simulink model "matlab_combined_demo_model"  (R2022b)
settings: Solver=ode4  StartTime=0.0  StopTime=inf  FixedStep=0.003  RelTol=1e-3
values from neighbouring files (symbols this model uses):
  A1 = 0    [load_quadrotor_simulink_combined_model.m]    (also in load_quadrotor_simulink_physics_model.m; load_quadtiltrotor_simulink_physics_model.m = 0.007)
  Apolar = 0    [load_quadrotor_simulink_combined_model.m]    (also in load_quadrotor_simulink_physics_model.m; load_quadtiltrotor_simulink_physics_model.m = 0.057)
  CD0 = 0    [load_quadrotor_simulink_combined_model.m]    (also in load_quadrotor_simulink_physics_model.m; load_quadtiltrotor_simulink_physics_model.m = 0.022)
  chord = 1    [load_quadrotor_simulink_combined_model.m]    (also in load_quadrotor_simulink_physics_model.m; load_quadtiltrotor_simulink_physics_model.m = 0.351342)
  CL0 = 0    [load_quadrotor_simulink_combined_model.m]    (also in load_quadrotor_simulink_physics_model.m; load_quadtiltrotor_simulink_physics_model.m = 0.38)
  CLa = 0    [load_quadrotor_simulink_combined_model.m]    (also in load_quadrotor_simulink_physics_model.m; load_quadtiltrotor_simulink_physics_model.m = 18.5)
  CLa_dot = 0    [load_quadrotor_simulink_combined_model.m]    (also in load_quadrotor_simulink_physics_model.m; load_quadtiltrotor_simulink_physics_model.m = 2.64)
  Clb = 0    [load_quadrotor_simulink_combined_model.m]    (also in load_quadrotor_simulink_physics_model.m; load_quadtiltrotor_simulink_physics_model.m)
  ClDa = 0    [load_quadrotor_simulink_combined_model.m]    (also in load_quadrotor_simulink_physics_model.m; load_quadtiltrotor_simulink_physics_model.m = 0.1695)
  CLDe = 0    [load_quadrotor_simulink_combined_model.m]    (also in load_quadrotor_simulink_physics_model.m; load_quadtiltrotor_simulink_physics_model.m)
  CLDf = 0    [load_quadrotor_simulink_combined_model.m]    (also in load_quadrotor_simulink_physics_model.m; load_quadtiltrotor_simulink_physics_model.m = 0.4)
  ClDr = 0    [load_quadrotor_simulink_combined_model.m]    (also in load_quadrotor_simulink_physics_model.m; load_quadtiltrotor_simulink_physics_model.m)
  Clp = 0    [load_quadrotor_simulink_combined_model.m]    (also in load_quadrotor_simulink_physics_model.m; load_quadtiltrotor_simulink_physics_model.m)
  CLq = 0    [load_quadrotor_simulink_combined_model.m]    (also in load_quadrotor_simulink_physics_model.m; load_quadtiltrotor_simulink_physics_model.m = 7.4)
  Clr = 0    [load_quadrotor_simulink_combined_model.m]    (also in load_quadrotor_simulink_physics_model.m; load_quadtiltrotor_simulink_physics_model.m)
  Cm0 = 0    [load_quadrotor_simulink_combined_model.m]    (also in load_quadrotor_simulink_physics_model.m; load_quadtiltrotor_simulink_physics_model.m)
  Cma = 0    [load_quadrotor_simulink_combined_model.m]    (also in load_quadrotor_simulink_physics_model.m; load_quadtiltrotor_simulink_physics_model.m)
  CmDe = 0    [load_quadrotor_simulink_combined_model.m]    (also in load_quadrotor_simulink_physics_model.m; load_quadtiltrotor_simulink_physics_model.m = -3.2)
  CmDf = 0    [load_quadrotor_simulink_combined_model.m]    (also in load_quadrotor_simulink_physics_model.m; load_quadtiltrotor_simulink_physics_model.m)
  Cmq = 0    [load_quadrotor_simulink_combined_model.m]    (also in load_quadrotor_simulink_physics_model.m; load_quadtiltrotor_simulink_physics_model.m)
  Cnb = 0    [load_quadrotor_simulink_combined_model.m]    (also in load_quadrotor_simulink_physics_model.m; load_quadtiltrotor_simulink_physics_model.m)
  CnDa = 0    [load_quadrotor_simulink_combined_model.m]    (also in load_quadrotor_simulink_physics_model.m; load_quadtiltrotor_simulink_physics_model.m = -0.023)
  CnDr = 0    [load_quadrotor_simulink_combined_model.m]    (also in load_quadrotor_simulink_physics_model.m; load_quadtiltrotor_simulink_physics_model.m)
  Cnp = 0    [load_quadrotor_simulink_combined_model.m]    (also in load_quadrotor_simulink_physics_model.m; load_quadtiltrotor_simulink_physics_model.m = -0.0889)
  Cnr = 0    [load_quadrotor_simulink_combined_model.m]    (also in load_quadrotor_simulink_physics_model.m; load_quadtiltrotor_simulink_physics_model.m = -0.19997)
  cross_section_area = 1    [load_quadrotor_simulink_combined_model.m]    (also in load_quadrotor_simulink_physics_model.m; load_quadtiltrotor_simulink_physics_model.m = 9.5)
  CYb = 0    [load_quadrotor_simulink_combined_model.m]    (also in load_quadrotor_simulink_physics_model.m; load_quadtiltrotor_simulink_physics_model.m = -1.098)
  CYDr = 0    [load_quadrotor_simulink_combined_model.m]    (also in load_quadrotor_simulink_physics_model.m; load_quadtiltrotor_simulink_physics_model.m = 0.143)
  drag_coeff_angular = -0.5    [load_quadrotor_simulink_combined_model.m]    (also in load_quadrotor_simulink_physics_model.m; load_quadtiltrotor_simulink_physics_model.m = 0.2)
  drag_coeff_linear = -0.5    [load_quadrotor_simulink_combined_model.m]    (also in load_quadrotor_simulink_physics_model.m; load_quadtiltrotor_simulink_physics_model.m = 0.2)
  elarm = 0    [load_quadrotor_simulink_combined_model.m]    (also in load_quadrotor_simulink_physics_model.m; load_quadtiltrotor_simulink_physics_model.m = 0.121)
  enable_FW_forces = 0    [load_quadrotor_simulink_combined_model.m]    (also in load_quadrotor_simulink_physics_model.m; load_quadtiltrotor_simulink_physics_model.m = 1)
  initial_rpy = [0, 0, 0]    [load_quadrotor_simulink_combined_model.m]    (also in load_quadrotor_simulink_physics_model.m; load_quadtiltrotor_simulink_physics_model.m)
  initial_xyz = [0, 0, -4]    [load_quadrotor_simulink_combined_model.m]    (also in load_quadrotor_simulink_physics_model.m; load_quadtiltrotor_simulink_physics_model.m = [2, 3, -4])
  mass = 1    [load_quadrotor_simulink_combined_model.m]    (also in load_quadrotor_simulink_physics_model.m; load_quadtiltrotor_simulink_physics_model.m = 10)
  span = 0    [load_quadrotor_simulink_combined_model.m]    (also in load_quadrotor_simulink_physics_model.m; load_quadtiltrotor_simulink_physics_model.m = 2.795)
libraries: aerolibutil x6, simulink x4, vrlib x4, sharedtransform x2, aerolibasang x2, shared6dof x1, matrix_library x1
(part 1 of 2)
settings Model: Creator=edufford  LastModifiedBy=edufford
settings DebuggingCC: UnconnectedInputMsg=warning  UnconnectedOutputMsg=warning  UnconnectedLineMsg=warning
settings ModelReferenceCC: EnableRefExpFcnMdlSchedulingChecks=on
settings RTWCC: DLArmComputeVersion=19.05

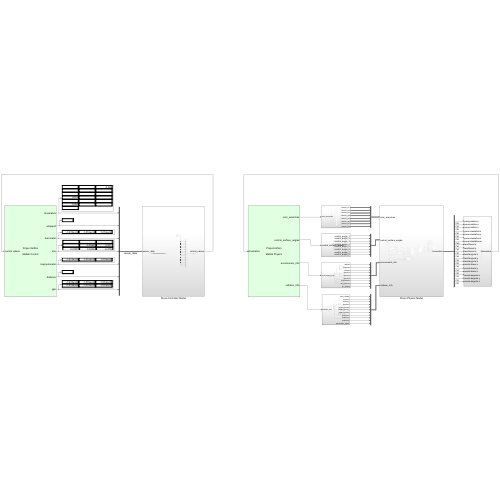
[thumbnail: Simulink's stored preview of the top-level diagram]
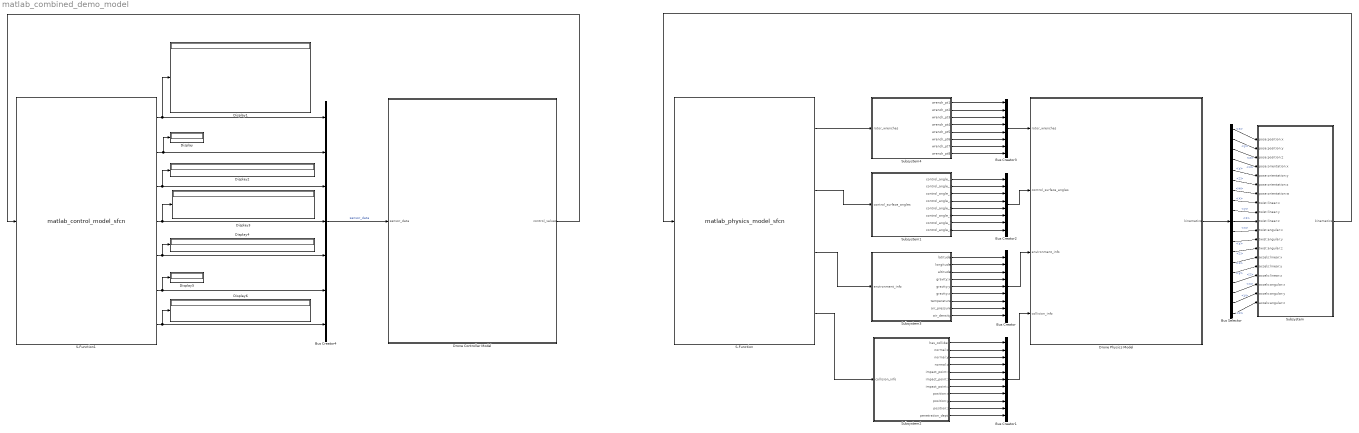
== system matlab_combined_demo_model ==
  Bus Creator : BusCreator  Inputs=9
  Bus Creator1 : BusCreator  Inputs=11
  Bus Creator2 : BusCreator  Inputs=8
  Bus Creator3 : BusCreator  Inputs=8
  Bus Creator4 : BusCreator  Inputs=7
  Bus Selector : BusSelector  OutputSignals=pose.position.x,pose.position.y,pose.position.z,pose.orientation.x,pose.orientation.y,pose.orientation.z,pose.orientation.w,twist.linear.x,twist.linear.y,twist.linear.z,twist.angular.x,twist.angular.y,twist.angular.z,accels.linear.x,accels.linear.y,accels.linear.z,accels.angular.x,accels.angular.y,accels.angular.z
  Display{,1..6} (7 alike) : Display
  Drone Controller Model : Subsystem
  Drone Physics Model : Subsystem
  S-Function : S-Function  Priority=10  FunctionName=matlab_physics_model_sfcn  Parameters=hostname,portnumber,timestep  SFunctionDeploymentMode=off  EnableBusSupport=off  mask{hostname=*, portnumber=8999, timestep=0.003}
      mask prompts: hostname "Host name:"; portnumber "Port number:"; timestep "AirSim time step:"
      mask Display:
      | disp("Project AirSim\n\n")
      | disp("\n\nMatlab Physics")
      | port_label('input',1,'kinematics')
      | port_label('output',1,'rotor_wrenches')
      | port_label('output',2,'control_surface_angles')
      | port_label('output',3,'environment_info')
      | port_label('output',4,'collision_info')
  S-Function1 : S-Function  Priority=20  FunctionName=matlab_control_model_sfcn  Parameters=hostname,portnumber,timestep  SFunctionDeploymentMode=off  EnableBusSupport=off  mask{hostname=*, portnumber=8998, timestep=0.003}
      mask prompts: hostname "Host name:"; portnumber "Port number:"; timestep "AirSim time step:"
      mask Display:
      | disp("Project AirSim\n\n")
      | disp("\n\nMatlab Control")
      | port_label('input',1,'control values')
      | port_label('output',1,'kinematics')
      | port_label('output',2,'airspeed')
      | port_label('output',3,'barometer')
      | port_label('output',4,'imu')
      | port_label('output',5,'magnetometer')
      | port_label('output',6,'distance')
      | port_label('output',7,'gps')
  Subsystem : Subsystem
  Subsystem1 : Subsystem
  Subsystem2 : Subsystem
  Subsystem3 : Subsystem
  Subsystem4 : Subsystem
  wires:
  Subsystem/1(kinematics) -> S-Function/1
  S-Function/4 -> Subsystem2/1(collision_info)
  Subsystem2/2(normal:x) -> Bus Creator1/2
  Subsystem2/5(impact_point:x) -> Bus Creator1/5
  Subsystem2/3(normal:y) -> Bus Creator1/3
  Subsystem2/4(normal:z) -> Bus Creator1/4
  Subsystem2/6(impact_point:y) -> Bus Creator1/6
  Subsystem2/7(impact_point:z) -> Bus Creator1/7
  Subsystem2/8(position:x) -> Bus Creator1/8
  Subsystem2/9(position:y) -> Bus Creator1/9
  Subsystem2/10(position:z) -> Bus Creator1/10
  Subsystem2/11(penetration_depth) -> Bus Creator1/11
  S-Function/3 -> Subsystem3/1(environment_info)
  Subsystem3/2(longitude) -> Bus Creator/2
  Subsystem3/3(altitude) -> Bus Creator/3
  Subsystem3/4(gravity:x) -> Bus Creator/4
  Subsystem3/5(gravity:y) -> Bus Creator/5
  Subsystem3/6(gravity:z) -> Bus Creator/6
  Subsystem3/7(temperature) -> Bus Creator/7
  Subsystem3/8(air_pressure) -> Bus Creator/8
  Subsystem3/9(air_density) -> Bus Creator/9
  Subsystem3/1(latitude) -> Bus Creator/1
  Bus Creator/1 -> Drone Physics Model/3(environment_info)
  Subsystem2/1(has_collided) -> Bus Creator1/1
  Bus Creator1/1 -> Drone Physics Model/4(collision_info)
  S-Function/1 -> Subsystem4/1(rotor_wrenches)
  Subsystem4/1(wrench_pt1) -> Bus Creator3/1
  Subsystem4/2(wrench_pt2) -> Bus Creator3/2
  Subsystem4/3(wrench_pt3) -> Bus Creator3/3
  Subsystem4/4(wrench_pt4) -> Bus Creator3/4
  Bus Creator3/1 -> Drone Physics Model/1(rotor_wrenches)
  Drone Physics Model/1(kinematics) -> Bus Selector/1
  Bus Selector/1 -> Subsystem/1(pose:position:x)  "<x>"
  Bus Selector/2 -> Subsystem/2(pose:position:y)  "<y>"
  Bus Selector/3 -> Subsystem/3(pose:position:z)  "<z>"
  Bus Selector/4 -> Subsystem/4(pose:orientation:x)  "<x>"
  Bus Selector/5 -> Subsystem/5(pose:orientation:y)  "<y>"
  Bus Selector/6 -> Subsystem/6(pose:orientation:z)  "<z>"
  Bus Selector/7 -> Subsystem/7(pose:orientation:w)  "<w>"
  Bus Selector/8 -> Subsystem/8(twist:linear:x)  "<x>"
  Bus Selector/9 -> Subsystem/9(twist:linear:y)  "<y>"
  Bus Selector/10 -> Subsystem/10(twist:linear:z)  "<z>"
  Bus Selector/11 -> Subsystem/11(twist:angular:x)  "<x>"
  Bus Selector/12 -> Subsystem/12(twist:angular:y)  "<y>"
  Bus Selector/13 -> Subsystem/13(twist:angular:z)  "<z>"
  Bus Selector/14 -> Subsystem/14(accels:linear:x)  "<x>"
  Bus Selector/15 -> Subsystem/15(accels:linear:y)  "<y>"
  Bus Selector/16 -> Subsystem/16(accels:linear:z)  "<z>"
  Bus Selector/17 -> Subsystem/17(accels:angular:x)  "<x>"
  Bus Selector/18 -> Subsystem/18(accels:angular:y)  "<y>"
  Bus Selector/19 -> Subsystem/19(accels:angular:z)  "<z>"
  Bus Creator2/1 -> Drone Physics Model/2(control_surface_angles)
  Subsystem1/1(control_angle_1) -> Bus Creator2/1
  Subsystem1/2(control_angle_2) -> Bus Creator2/2
  Subsystem1/3(control_angle_3) -> Bus Creator2/3
  S-Function/2 -> Subsystem1/1(control_surface_angles)
  Subsystem4/5(wrench_pt5) -> Bus Creator3/5
  Subsystem4/6(wrench_pt6) -> Bus Creator3/6
  Subsystem4/7(wrench_pt7) -> Bus Creator3/7
  Subsystem4/8(wrench_pt8) -> Bus Creator3/8
  Subsystem1/4(control_angle_4) -> Bus Creator2/4
  Subsystem1/5(control_angle_5) -> Bus Creator2/5
  Subsystem1/6(control_angle_6) -> Bus Creator2/6
  Subsystem1/7(control_angle_7) -> Bus Creator2/7
  Subsystem1/8(control_angle_8) -> Bus Creator2/8
  Drone Controller Model/1(control_values) -> S-Function1/1
  S-Function1/1 -> Display1/1, Bus Creator4/1
  S-Function1/2 -> Bus Creator4/2, Display/1
  S-Function1/3 -> Display2/1, Bus Creator4/3
  S-Function1/4 -> Display3/1, Bus Creator4/4
  S-Function1/5 -> Display4/1, Bus Creator4/5
  S-Function1/6 -> Display5/1, Bus Creator4/6
  S-Function1/7 -> Display6/1, Bus Creator4/7
  Bus Creator4/1 -> Drone Controller Model/1(sensor_data)  "sensor_data"

== system matlab_combined_demo_model/Drone Controller Model ==
  sensor_data : Inport
  Mux : Mux  Inputs=16
  Repeating Sequence : simulink/Sources/Repeating Sequence  rep_seq_t=[0 5 10]  rep_seq_y=[0 1 0]
  Terminator : Terminator
  control_values : Outport
  wires:
  Repeating Sequence/1 -> Mux/1, Mux/2, Mux/3, Mux/7, Mux/8, Mux/9, Mux/10, Mux/11, Mux/14, Mux/15, Mux/16, Mux/13, Mux/12, Mux/6, Mux/5, Mux/4
  Mux/1 -> control_values/1
  sensor_data/1 -> Terminator/1

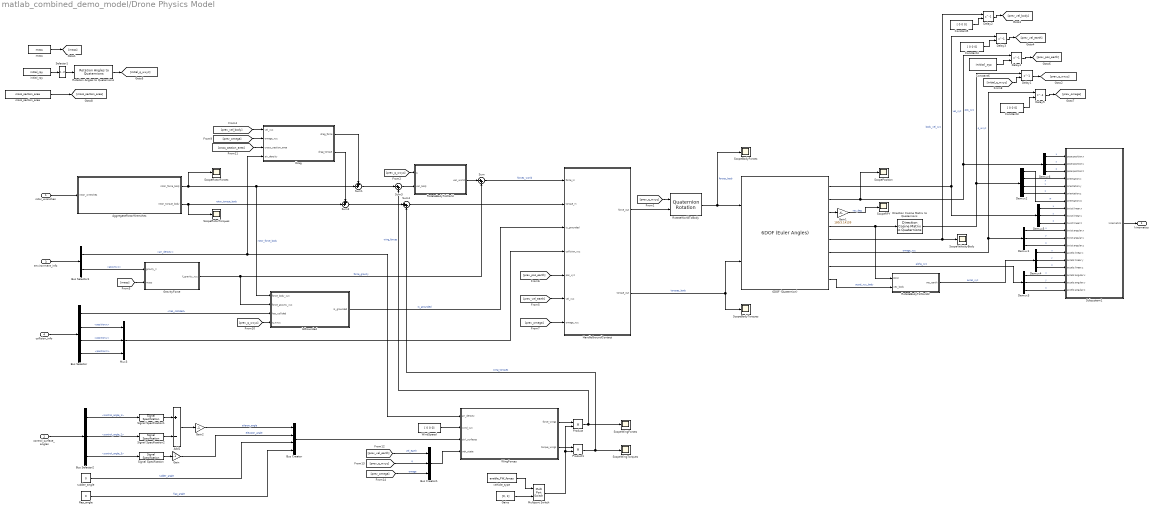
== system matlab_combined_demo_model/Drone Physics Model ==
  rotor_wrenches : Inport
  control_surface_angles : Inport  Port=2
  environment_info : Inport  Port=3
  collision_info : Inport  Port=4
  6DOF (Quaternion) : shared6dof/6DOF (Euler Angles)  units=Metric (MKS)  mtype=Fixed  rep=Quaternion  xme_0=initial_xyz  Vm_0=initial_vel_xyz  eul_0=initial_rpy  pm_0=initial_ang_rot_xyz  mass_0=mass  mass_e=0.5  mass_f=2.0  inertia=inertia  inertia_e=eye(3)  inertia_f=2*eye(3)  k_quat=1.0  vre_flag=on  abi_flag=off  aMode=0  xme_statename=''  Vm_statename=''  eul_statename=''  quat_statename=''  pm_statename=''  mass_statename=''
  Add1 : Sum  Inputs=+-
  AggregateRotorWrenches : Subsystem
  Bus Creator : BusCreator  Inputs=4
  Bus Creator1 : BusCreator  Inputs=3
  Bus Selector : BusSelector  OutputSignals=has_collided,position:x,position:y,position:z
  Bus Selector1 : BusSelector  OutputSignals=air_density,gravity:z
  Bus Selector2 : BusSelector  OutputSignals=control_angle_1,control_angle_2,control_angle_3
  Constant3 : Constant  Value=[ 0 0 0]
      settings: AttributesFormatString=%<Value>
  Constant4 : Constant  Value=[ 0 0 0]
      settings: AttributesFormatString=%<Value>
  Constant5 : Constant  Value=[ 0 0 0]
      settings: AttributesFormatString=%<Value>
  Constant6 : Constant  Value=initial_xyz
      settings: AttributesFormatString=%<Value>
  Delay{1..5} (5 alike) : Delay  DelayLength=1  InitialConditionSource=Input port  InitialCondition=0
      settings: InputPortMap=u0,p4
  Demux{1,3..6} (5 alike) : Demux  Outputs=3
  Demux2 : Demux
  Direction Cosine Matrix to Quaternions : sharedtransform/Direction Cosine Matrix  to Quaternions  aMode=0  action=None  tolerance=eps(2)
  Drag : Subsystem
  Gain : Gain  Gain=-1
  Gain1 : Gain  Gain=180/3.14159
  Gain2 : Gain  Gain=-1
  Gains : Constant  Value=[0, 1]
  GravityForce : Subsystem
  HandleGroundContact : Subsystem
  IsGrounded : Subsystem
  Multiport Switch : MultiPortSwitch  DataPortOrder=Zero-based contiguous  Inputs=1  zeroidx=on  SaturateOnIntegerOverflow=off  InputSameDT=off
  Mux3 : Mux  Inputs=3
  Product : Product
  Product1 : Product
  RotateBodyToWorld : Subsystem
  RotateBodyToWorld2 : Subsystem
  RotateWorldToBody : aerolibutil/Quaternion Rotation
  Rotation Angles to Quaternions : sharedtransform/Rotation Angles to Quaternions  rotationOrder=ZYX  aMode=aMode
  ScopeBodyForces : Scope
  ScopeBodyTorques : Scope
  ScopePosition : Scope
  ScopeRPY : Scope
  ScopeRotorForces : Scope
  ScopeRotorTorques : Scope
  ScopeVelocityBody : Scope
  ScopeWingForces : Scope
  ScopeWingTorques : Scope
  Selector1 : Selector  InputPortWidth=3  IndexOptions=Index vector (dialog)  Indices=[3 2 1]  OutputSizes=1
  Signal Specification : SignalSpecification  Unit=rad
  Signal Specification1 : SignalSpecification  Unit=rad
  Signal Specification2 : SignalSpecification  Unit=rad
  Subsystem1 : Subsystem
  Sum : Sum  Inputs=|++
  Sum1 : Sum  Inputs=++|
  Sum2 : Sum  Inputs=++|
  Sum3 : Sum  Inputs=|++
  Sum4 : Sum  Inputs=|++
  WindSpeed : Constant  Value=[ 0 0 0]
      settings: AttributesFormatString=%<Value>
  WingForces : Subsystem
  cross_section_area : Constant  Value=cross_section_area
  flap_angle : Constant  Value=0
  initial_rpy : Constant  Value=initial_rpy
  mass : Constant  Value=mass
  rudder_angle : Constant  Value=0
  vehicle_type : Constant  Value=enable_FW_forces
  kinematics : Outport
  wires:
  collision_info/1 -> Bus Selector/1
  environment_info/1 -> Bus Selector1/1
  rotor_wrenches/1 -> AggregateRotorWrenches/1(rotor_wrenches)
  Subsystem1/1(kinematics) -> kinematics/1
  Demux2/2 -> Subsystem1/4(orientation:x)  "x"
  Demux2/3 -> Subsystem1/5(orientation:y)  "y"
  Demux2/4 -> Subsystem1/6(orientation:z)  "z"
  Bus Selector/1 -> IsGrounded/3(has_collided)  "<has_collided>"
  Demux2/1 -> Subsystem1/7(orientation:w)  "w"
  Demux1/1 -> Subsystem1/11(twist:angular:x)  "x"
  Demux1/2 -> Subsystem1/12(twist:angular:y)  "y"
  Demux1/3 -> Subsystem1/13(twist:angular:z)  "z"
  Demux3/1 -> Subsystem1/17(accels:angular:x)  "x"
  Demux3/2 -> Subsystem1/18(accels:angular:y)  "y"
  Demux3/3 -> Subsystem1/19(accels:angular:z)  "z"
  initial_rpy/1 -> Selector1/1
  IsGrounded/1(is_grounded) -> HandleGroundContact/3(is_grounded)  "is_grounded"
  Bus Selector/4 -> Mux3/3  "<position:z>"
  [initial_q_wxyz] -> Delay1/2
  Demux4/1 -> Subsystem1/14(accels:linear:x)  "x"
  Demux4/2 -> Subsystem1/15(accels:linear:y)  "y"
  Demux4/3 -> Subsystem1/16(accels:linear:z)  "z"
  Demux5/1 -> Subsystem1/8(twist:linear:x)  "x"
  Demux5/2 -> Subsystem1/9(twist:linear:y)  "y"
  Demux5/3 -> Subsystem1/10(twist:linear:z)  "z"
  Demux6/1 -> Subsystem1/1(pose:position:x)  "x"
  Demux6/2 -> Subsystem1/2(pose:position:y)  "y"
  Demux6/3 -> Subsystem1/3(pose:position:z)  "z"
  6DOF (Quaternion)/1 -> Demux5/1, Delay3/1  "vel_xyz"
  6DOF (Quaternion)/3 -> Gain1/1
  6DOF (Quaternion)/4 -> RotateBodyToWorld2/1(DCM), Direction Cosine Matrix to Quaternions/1
  6DOF (Quaternion)/7 -> Demux3/1  "alpha_xyz"
  mass/1 -> [mass]
  6DOF (Quaternion)/2 -> Demux6/1, Delay4/1, ScopePosition/1  "pos_xyz"
  Direction Cosine Matrix to Quaternions/1 -> Demux2/1, Delay1/1  "q_wxyz"
  6DOF (Quaternion)/8 -> RotateBodyToWorld2/2(vec_body)  "accel_xyz_body"
  RotateBodyToWorld2/1(vec_earth) -> Demux4/1  "accel_xyz"
  Rotation Angles to Quaternions/1 -> [initial_q_wxyz]
  Selector1/1 -> Rotation Angles to Quaternions/1
  Delay1/1 -> [prev_q_wxyz]
  [prev_q_wxyz] -> RotateWorldToBody/1
  Delay2/1 -> [prev_vel_body]
  [prev_vel_body] -> Drag/1(vel_xyz)
  Delay3/1 -> [prev_vel_earth]
  [prev_vel_earth] -> HandleGroundContact/6(vel_xyz)
  Delay4/1 -> [prev_pos_earth]
  [prev_pos_earth] -> HandleGroundContact/5(pos_xyz)
  Delay5/1 -> [prev_omega]
  [prev_omega] -> HandleGroundContact/7(omega_xyz)
  Bus Selector/3 -> Mux3/2  "<position:y>"
  Bus Selector/2 -> Mux3/1  "<position:x>"
  Mux3/1 -> HandleGroundContact/4(collision_xyz)
  GravityForce/1(f_gravity_xyz) -> IsGrounded/2(force_gravity_xyz), Sum/2  "force_gravity"
  Bus Selector1/2 -> GravityForce/1(gravity_z)  "<gravity:z>"
  [mass] -> GravityForce/2(mass)
  [prev_q_wxyz] -> RotateBodyToWorld/1(q)
  RotateBodyToWorld/1(vec_world) -> Sum/1
  [prev_omega] -> Drag/2(omega_xyz)
  HandleGroundContact/2(torque_out) -> 6DOF (Quaternion)/2, ScopeBodyTorques/1  "torques_body"
  RotateWorldToBody/1 -> 6DOF (Quaternion)/1, ScopeBodyForces/1  "forces_body"
  HandleGroundContact/1(force_out) -> RotateWorldToBody/2
  Sum/1 -> HandleGroundContact/1(force_in)  "forces_world"
  Drag/2(drag_torque) -> Sum2/1
  Drag/1(drag_force) -> Sum1/1
  Sum1/1 -> Sum3/1
  [prev_q_wxyz] -> IsGrounded/4(q_wxyz)
  Sum4/1 -> HandleGroundContact/2(torque_in)
  Gain1/1 -> ScopeRPY/1  "rpy_deg"
  Bus Selector1/1 -> Drag/4(air_density), WingForces/1(air_density)  "<air_density>"
  [cross_section_area] -> Drag/3(cross_section_area)
  control_surface_angles/1 -> Bus Selector2/1
  Bus Selector2/1 -> Signal Specification1/1  "<control_angle_1>"
  Bus Selector2/2 -> Signal Specification2/1  "<control_angle_2>"
  Bus Selector2/3 -> Signal Specification/1  "<control_angle_3>"
  Signal Specification1/1 -> Add1/1
  Signal Specification2/1 -> Add1/2
  flap_angle/1 -> Bus Creator/4  "flap_angle"
  Sum3/1 -> RotateBodyToWorld/2(vec_body)
  Sum2/1 -> Sum4/1
  Constant3/1 -> Delay5/2
  Constant4/1 -> Delay3/2
  Constant5/1 -> Delay2/2
  Constant6/1 -> Delay4/2
  Bus Creator/1 -> WingForces/3(ctrl_surfaces)
  [prev_vel_earth] -> Bus Creator1/1  "vel_earth"
  [prev_q_wxyz] -> Bus Creator1/2  "q"
  [prev_omega] -> Bus Creator1/3  "omega"
  Bus Creator1/1 -> WingForces/4(veh_state)
  WindSpeed/1 -> WingForces/2(wind_xyz)
  Signal Specification/1 -> Gain/1
  Add1/1 -> Gain2/1
  6DOF (Quaternion)/6 -> Demux1/1, Delay5/1  "omega_xyz"
  6DOF (Quaternion)/5 -> ScopeVelocityBody/1, Delay2/1  "body_vel_xyz"
  rudder_angle/1 -> Bus Creator/3  "rudder_angle"
  Gain/1 -> Bus Creator/2  "elevator_angle"
  Gain2/1 -> Bus Creator/1  "aileron_angle"
  cross_section_area/1 -> [cross_section_area]
  vehicle_type/1 -> Multiport Switch/1
  Gains/1 -> Multiport Switch/2
  AggregateRotorWrenches/2(rotor_torque_body) -> Sum2/2, ScopeRotorTorques/1  "rotor_torque_body"
  AggregateRotorWrenches/1(rotor_force_body) -> Sum1/2, IsGrounded/1(force_body_xyz), ScopeRotorForces/1  "rotor_force_body"
  WingForces/1(force_wings) -> Product/1
  Product/1 -> Sum3/2, ScopeWingForces/1  "wing_forces"
  WingForces/2(torque_wings) -> Product1/1
  Product1/1 -> ScopeWingTorques/1, Sum4/2  "wing_torques"
  Multiport Switch/1 -> Product1/2, Product/2

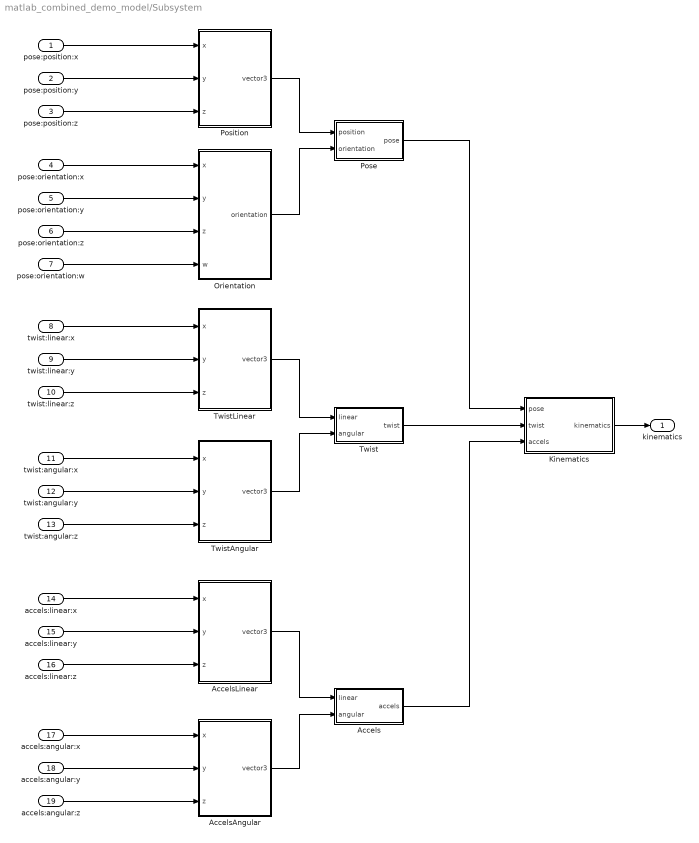
== system matlab_combined_demo_model/Subsystem ==
  pose:position:x : Inport
  pose:position:y : Inport  Port=2
  pose:position:z : Inport  Port=3
  pose:orientation:x : Inport  Port=4
  pose:orientation:y : Inport  Port=5
  pose:orientation:z : Inport  Port=6
  pose:orientation:w : Inport  Port=7
  twist:linear:x : Inport  Port=8
  twist:linear:y : Inport  Port=9
  twist:linear:z : Inport  Port=10
  twist:angular:x : Inport  Port=11
  twist:angular:y : Inport  Port=12
  twist:angular:z : Inport  Port=13
  accels:linear:x : Inport  Port=14
  accels:linear:y : Inport  Port=15
  accels:linear:z : Inport  Port=16
  accels:angular:x : Inport  Port=17
  accels:angular:y : Inport  Port=18
  accels:angular:z : Inport  Port=19
  Accels : Subsystem
  AccelsAngular : Subsystem
  AccelsLinear : Subsystem
  Kinematics : Subsystem
  Orientation : Subsystem
  Pose : Subsystem
  Position : Subsystem
  Twist : Subsystem
  TwistAngular : Subsystem
  TwistLinear : Subsystem
  kinematics : Outport
  wires:
  AccelsLinear/1(vector3) -> Accels/1(linear)
  AccelsAngular/1(vector3) -> Accels/2(angular)
  accels:angular:x/1 -> AccelsAngular/1(x)
  accels:angular:y/1 -> AccelsAngular/2(y)
  accels:angular:z/1 -> AccelsAngular/3(z)
  accels:linear:z/1 -> AccelsLinear/3(z)
  accels:linear:y/1 -> AccelsLinear/2(y)
  accels:linear:x/1 -> AccelsLinear/1(x)
  pose:orientation:x/1 -> Orientation/1(x)
  pose:orientation:y/1 -> Orientation/2(y)
  pose:position:y/1 -> Position/2(y)
  pose:position:x/1 -> Position/1(x)
  pose:orientation:z/1 -> Orientation/3(z)
  pose:position:z/1 -> Position/3(z)
  pose:orientation:w/1 -> Orientation/4(w)
  Position/1(vector3) -> Pose/1(position)
  Orientation/1(orientation) -> Pose/2(orientation)
  twist:linear:x/1 -> TwistLinear/1(x)
  twist:linear:y/1 -> TwistLinear/2(y)
  twist:linear:z/1 -> TwistLinear/3(z)
  twist:angular:x/1 -> TwistAngular/1(x)
  twist:angular:y/1 -> TwistAngular/2(y)
  twist:angular:z/1 -> TwistAngular/3(z)
  TwistLinear/1(vector3) -> Twist/1(linear)
  TwistAngular/1(vector3) -> Twist/2(angular)
  Pose/1(pose) -> Kinematics/1(pose)
  Twist/1(twist) -> Kinematics/2(twist)
  Accels/1(accels) -> Kinematics/3(accels)
  Kinematics/1(kinematics) -> kinematics/1

== system matlab_combined_demo_model/Subsystem1 ==
  control_surface_angles : Inport
  Demux : Demux  Outputs=8
  control_angle_1 : Outport
  control_angle_2 : Outport  Port=2
  control_angle_3 : Outport  Port=3
  control_angle_4 : Outport  Port=4
  control_angle_5 : Outport  Port=5
  control_angle_6 : Outport  Port=6
  control_angle_7 : Outport  Port=7
  control_angle_8 : Outport  Port=8
  wires:
  control_surface_angles/1 -> Demux/1
  Demux/8 -> control_angle_8/1  "control_angle_8"
  Demux/7 -> control_angle_7/1  "control_angle_7"
  Demux/6 -> control_angle_6/1  "control_angle_6"
  Demux/5 -> control_angle_5/1  "control_angle_5"
  Demux/1 -> control_angle_1/1  "control_angle_1"
  Demux/2 -> control_angle_2/1  "control_angle_2"
  Demux/3 -> control_angle_3/1  "control_angle_3"
  Demux/4 -> control_angle_4/1  "control_angle_4"

== system matlab_combined_demo_model/Subsystem2 ==
  collision_info : Inport
  Demux : Demux  Outputs=5
  Demux1 : Demux  Outputs=3
  Demux2 : Demux  Outputs=3
  Demux3 : Demux  Outputs=3
  has_collided : Outport  PortDimensions=1
  normal:x : Outport  Port=2
  normal:y : Outport  Port=3
  normal:z : Outport  Port=4
  impact_point:x : Outport  Port=5
  impact_point:y : Outport  Port=6
  impact_point:z : Outport  Port=7
  position:x : Outport  Port=8
  position:y : Outport  Port=9
  position:z : Outport  Port=10
  penetration_depth : Outport  Port=11  PortDimensions=1
  wires:
  Demux/4 -> Demux3/1  "position"
  Demux3/3 -> position:z/1  "position:z"
  Demux/1 -> has_collided/1  "has_collided"
  Demux/3 -> Demux2/1  "impact_point"
  Demux1/2 -> normal:y/1  "normal:y"
  Demux/2 -> Demux1/1  "normal"
  Demux3/2 -> position:y/1  "position:y"
  Demux2/2 -> impact_point:y/1  "impact_point:y"
  collision_info/1 -> Demux/1
  Demux2/1 -> impact_point:x/1  "impact_point:x"
  Demux2/3 -> impact_point:z/1  "impact_point:z"
  Demux3/1 -> position:x/1  "position:x"
  Demux/5 -> penetration_depth/1  "penetration_depth"
  Demux1/3 -> normal:z/1  "normal:z"
  Demux1/1 -> normal:x/1  "normal:x"

== system matlab_combined_demo_model/Subsystem3 ==
  environment_info : Inport
  Demux : Demux  Outputs=5
  Demux1 : Demux  Outputs=3
  Demux3 : Demux  Outputs=3
  latitude : Outport  PortDimensions=1
  longitude : Outport  Port=2  PortDimensions=1
  altitude : Outport  Port=3  PortDimensions=1
  gravity:x : Outport  Port=4  PortDimensions=1
  gravity:y : Outport  Port=5  PortDimensions=1
  gravity:z : Outport  Port=6  PortDimensions=1
  temperature : Outport  Port=7  PortDimensions=1
  air_pressure : Outport  Port=8  PortDimensions=1
  air_density : Outport  Port=9  PortDimensions=1
  wires:
  Demux1/2 -> longitude/1  "longitude"
  Demux/4 -> air_pressure/1  "air_pressure"
  Demux3/1 -> gravity:x/1  "gravity:x"
  Demux/5 -> air_density/1  "air_density"
  Demux3/2 -> gravity:y/1  "gravity:y"
  Demux1/1 -> latitude/1  "latitude"
  environment_info/1 -> Demux/1
  Demux/2 -> Demux3/1  "gravity"
  Demux/3 -> temperature/1  "temperature"
  Demux3/3 -> gravity:z/1  "gravity:z"
  Demux1/3 -> altitude/1  "altitude"
  Demux/1 -> Demux1/1  "geopoint"

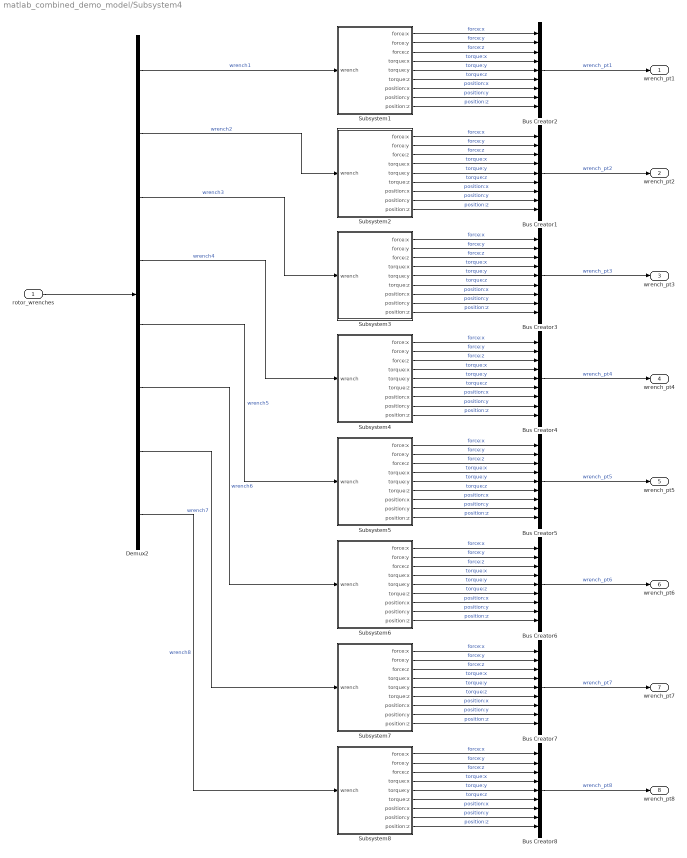
== system matlab_combined_demo_model/Subsystem4 ==
  rotor_wrenches : Inport
  Bus Creator{1..8} (8 alike) : BusCreator  Inputs=9
  Demux2 : Demux  Outputs=8
  Subsystem1 : Subsystem
  Subsystem2 : Subsystem
  Subsystem3 : Subsystem
  Subsystem4 : Subsystem
  Subsystem5 : Subsystem
  Subsystem6 : Subsystem
  Subsystem7 : Subsystem
  Subsystem8 : Subsystem
  wrench_pt1 : Outport
  wrench_pt2 : Outport  Port=2
  wrench_pt3 : Outport  Port=3
  wrench_pt4 : Outport  Port=4
  wrench_pt5 : Outport  Port=5
  wrench_pt6 : Outport  Port=6
  wrench_pt7 : Outport  Port=7
  wrench_pt8 : Outport  Port=8
  wires:
  Demux2/1 -> Subsystem1/1(wrench)  "wrench1"
  Bus Creator2/1 -> wrench_pt1/1  "wrench_pt1"
  rotor_wrenches/1 -> Demux2/1
  Bus Creator1/1 -> wrench_pt2/1  "wrench_pt2"
  Subsystem2/8(position:y) -> Bus Creator1/8  "position:y"
  Subsystem2/4(torque:x) -> Bus Creator1/4  "torque:x"
  Subsystem2/6(torque:z) -> Bus Creator1/6  "torque:z"
  Subsystem2/9(position:z) -> Bus Creator1/9  "position:z"
  Subsystem2/7(position:x) -> Bus Creator1/7  "position:x"
  Subsystem2/1(force:x) -> Bus Creator1/1  "force:x"
  Subsystem2/5(torque:y) -> Bus Creator1/5  "torque:y"
  Subsystem2/3(force:z) -> Bus Creator1/3  "force:z"
  Subsystem2/2(force:y) -> Bus Creator1/2  "force:y"
  Demux2/2 -> Subsystem2/1(wrench)  "wrench2"
  Bus Creator3/1 -> wrench_pt3/1  "wrench_pt3"
  Bus Creator4/1 -> wrench_pt4/1  "wrench_pt4"
  Demux2/4 -> Subsystem4/1(wrench)  "wrench4"
  Subsystem1/3(force:z) -> Bus Creator2/3  "force:z"
  Subsystem1/2(force:y) -> Bus Creator2/2  "force:y"
  Subsystem1/7(position:x) -> Bus Creator2/7  "position:x"
  Subsystem1/1(force:x) -> Bus Creator2/1  "force:x"
  Subsystem1/8(position:y) -> Bus Creator2/8  "position:y"
  Subsystem1/5(torque:y) -> Bus Creator2/5  "torque:y"
  Subsystem1/9(position:z) -> Bus Creator2/9  "position:z"
  Subsystem1/6(torque:z) -> Bus Creator2/6  "torque:z"
  Subsystem1/4(torque:x) -> Bus Creator2/4  "torque:x"
  Subsystem3/3(force:z) -> Bus Creator3/3  "force:z"
  Subsystem3/2(force:y) -> Bus Creator3/2  "force:y"
  Subsystem3/7(position:x) -> Bus Creator3/7  "position:x"
  Subsystem3/1(force:x) -> Bus Creator3/1  "force:x"
  Subsystem3/8(position:y) -> Bus Creator3/8  "position:y"
  Subsystem3/5(torque:y) -> Bus Creator3/5  "torque:y"
  Subsystem3/9(position:z) -> Bus Creator3/9  "position:z"
  Subsystem3/6(torque:z) -> Bus Creator3/6  "torque:z"
  Subsystem3/4(torque:x) -> Bus Creator3/4  "torque:x"
  Subsystem4/3(force:z) -> Bus Creator4/3  "force:z"
  Subsystem4/2(force:y) -> Bus Creator4/2  "force:y"
  Subsystem4/7(position:x) -> Bus Creator4/7  "position:x"
  Subsystem4/1(force:x) -> Bus Creator4/1  "force:x"
  Subsystem4/8(position:y) -> Bus Creator4/8  "position:y"
  Subsystem4/5(torque:y) -> Bus Creator4/5  "torque:y"
  Subsystem4/9(position:z) -> Bus Creator4/9  "position:z"
  Subsystem4/6(torque:z) -> Bus Creator4/6  "torque:z"
  Subsystem4/4(torque:x) -> Bus Creator4/4  "torque:x"
  Demux2/3 -> Subsystem3/1(wrench)  "wrench3"
  Demux2/8 -> Subsystem8/1(wrench)  "wrench8"
  Demux2/7 -> Subsystem7/1(wrench)  "wrench7"
  Demux2/6 -> Subsystem6/1(wrench)  "wrench6"
  Demux2/5 -> Subsystem5/1(wrench)  "wrench5"
  Subsystem5/9(position:z) -> Bus Creator5/9  "position:z"
  Subsystem5/7(position:x) -> Bus Creator5/7  "position:x"
  Subsystem5/5(torque:y) -> Bus Creator5/5  "torque:y"
  Bus Creator5/1 -> wrench_pt5/1  "wrench_pt5"
  Subsystem5/8(position:y) -> Bus Creator5/8  "position:y"
  Subsystem5/4(torque:x) -> Bus Creator5/4  "torque:x"
  Subsystem5/3(force:z) -> Bus Creator5/3  "force:z"
  Subsystem5/6(torque:z) -> Bus Creator5/6  "torque:z"
  Subsystem5/2(force:y) -> Bus Creator5/2  "force:y"
  Subsystem5/1(force:x) -> Bus Creator5/1  "force:x"
  Subsystem6/4(torque:x) -> Bus Creator6/4  "torque:x"
  Subsystem6/8(position:y) -> Bus Creator6/8  "position:y"
  Subsystem6/3(force:z) -> Bus Creator6/3  "force:z"
  Subsystem6/6(torque:z) -> Bus Creator6/6  "torque:z"
  Subsystem6/2(force:y) -> Bus Creator6/2  "force:y"
  Bus Creator6/1 -> wrench_pt6/1  "wrench_pt6"
  Subsystem6/7(position:x) -> Bus Creator6/7  "position:x"
  Subsystem6/5(torque:y) -> Bus Creator6/5  "torque:y"
  Subsystem6/9(position:z) -> Bus Creator6/9  "position:z"
  Subsystem6/1(force:x) -> Bus Creator6/1  "force:x"
  Subsystem7/1(force:x) -> Bus Creator7/1  "force:x"
  Subsystem7/9(position:z) -> Bus Creator7/9  "position:z"
  Subsystem7/5(torque:y) -> Bus Creator7/5  "torque:y"
  Subsystem7/7(position:x) -> Bus Creator7/7  "position:x"
  Bus Creator7/1 -> wrench_pt7/1  "wrench_pt7"
  Subsystem7/2(force:y) -> Bus Creator7/2  "force:y"
  Subsystem7/6(torque:z) -> Bus Creator7/6  "torque:z"
  Subsystem7/3(force:z) -> Bus Creator7/3  "force:z"
  Subsystem7/8(position:y) -> Bus Creator7/8  "position:y"
  Subsystem7/4(torque:x) -> Bus Creator7/4  "torque:x"
  Subsystem8/8(position:y) -> Bus Creator8/8  "position:y"
  Subsystem8/3(force:z) -> Bus Creator8/3  "force:z"
  Subsystem8/4(torque:x) -> Bus Creator8/4  "torque:x"
  Subsystem8/2(force:y) -> Bus Creator8/2  "force:y"
  Subsystem8/6(torque:z) -> Bus Creator8/6  "torque:z"
  Subsystem8/5(torque:y) -> Bus Creator8/5  "torque:y"
  Subsystem8/9(position:z) -> Bus Creator8/9  "position:z"
  Subsystem8/7(position:x) -> Bus Creator8/7  "position:x"
  Bus Creator8/1 -> wrench_pt8/1  "wrench_pt8"
  Subsystem8/1(force:x) -> Bus Creator8/1  "force:x"

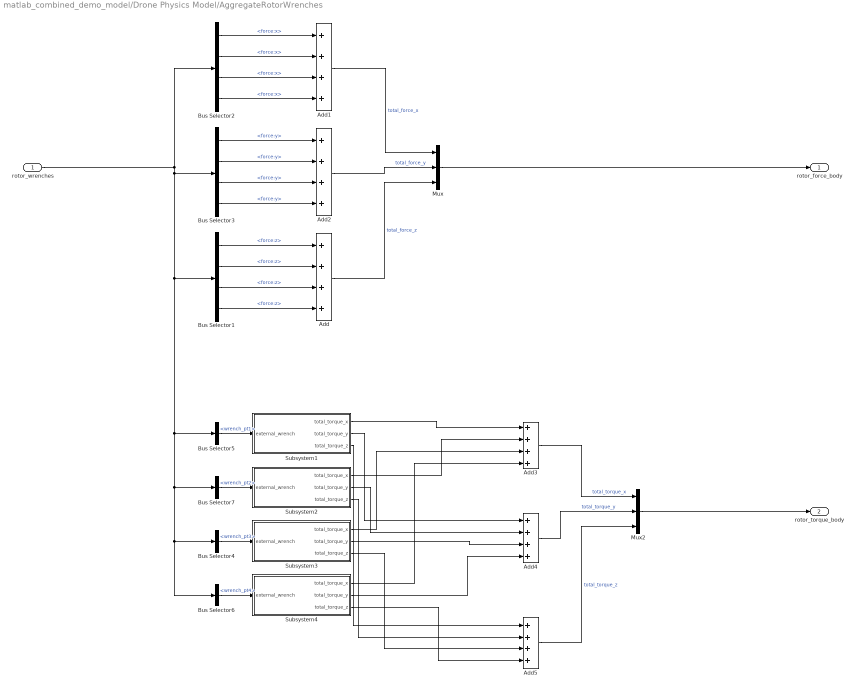
== system matlab_combined_demo_model/Drone Physics Model/AggregateRotorWrenches ==
  rotor_wrenches : Inport
  Add{,1..5} (6 alike) : Sum  Inputs=++++
  Bus Selector1 : BusSelector  OutputSignals=wrench_pt1.force:z,wrench_pt2.force:z,wrench_pt3.force:z,wrench_pt4.force:z
  Bus Selector2 : BusSelector  OutputSignals=wrench_pt1.force:x,wrench_pt2.force:x,wrench_pt3.force:x,wrench_pt4.force:x
  Bus Selector3 : BusSelector  OutputSignals=wrench_pt1.force:y,wrench_pt2.force:y,wrench_pt3.force:y,wrench_pt4.force:y
  Bus Selector4 : BusSelector  OutputSignals=wrench_pt3
  Bus Selector5 : BusSelector  OutputSignals=wrench_pt1
  Bus Selector6 : BusSelector  OutputSignals=wrench_pt4
  Bus Selector7 : BusSelector  OutputSignals=wrench_pt2
  Mux : Mux  Inputs=3
  Mux2 : Mux  Inputs=3
  Subsystem1 : Subsystem
  Subsystem2 : Subsystem
  Subsystem3 : Subsystem
  Subsystem4 : Subsystem
  rotor_force_body : Outport  PortDimensions=[3]
  rotor_torque_body : Outport  Port=2
  wires:
  Bus Selector1/1 -> Add/1  "<force:z>"
  Bus Selector1/2 -> Add/2  "<force:z>"
  Bus Selector1/3 -> Add/3  "<force:z>"
  Bus Selector1/4 -> Add/4  "<force:z>"
  Bus Selector2/1 -> Add1/1  "<force:x>"
  Bus Selector2/2 -> Add1/2  "<force:x>"
  Bus Selector2/3 -> Add1/3  "<force:x>"
  Bus Selector2/4 -> Add1/4  "<force:x>"
  Bus Selector3/2 -> Add2/2  "<force:y>"
  Bus Selector3/1 -> Add2/1  "<force:y>"
  Bus Selector3/3 -> Add2/3  "<force:y>"
  Bus Selector3/4 -> Add2/4  "<force:y>"
  Add1/1 -> Mux/1  "total_force_x"
  Add2/1 -> Mux/2  "total_force_y"
  Add/1 -> Mux/3  "total_force_z"
  Bus Selector5/1 -> Subsystem1/1(external_wrench)  "<wrench_pt1>"
  Bus Selector7/1 -> Subsystem2/1(external_wrench)  "<wrench_pt2>"
  Bus Selector4/1 -> Subsystem3/1(external_wrench)  "<wrench_pt3>"
  Bus Selector6/1 -> Subsystem4/1(external_wrench)  "<wrench_pt4>"
  rotor_wrenches/1 -> Bus Selector6/1, Bus Selector4/1, Bus Selector7/1, Bus Selector5/1, Bus Selector1/1, Bus Selector3/1, Bus Selector2/1
  Subsystem1/1(total_torque_x) -> Add3/1
  Subsystem2/1(total_torque_x) -> Add3/2
  Subsystem3/1(total_torque_x) -> Add3/3
  Subsystem4/1(total_torque_x) -> Add3/4
  Subsystem1/2(total_torque_y) -> Add4/1
  Subsystem2/2(total_torque_y) -> Add4/2
  Subsystem3/2(total_torque_y) -> Add4/3
  Subsystem4/2(total_torque_y) -> Add4/4
  Subsystem1/3(total_torque_z) -> Add5/1
  Subsystem2/3(total_torque_z) -> Add5/2
  Subsystem3/3(total_torque_z) -> Add5/3
  Subsystem4/3(total_torque_z) -> Add5/4
  Add3/1 -> Mux2/1  "total_torque_x"
  Add4/1 -> Mux2/2  "total_torque_y"
  Add5/1 -> Mux2/3  "total_torque_z"
  Mux2/1 -> rotor_torque_body/1
  Mux/1 -> rotor_force_body/1

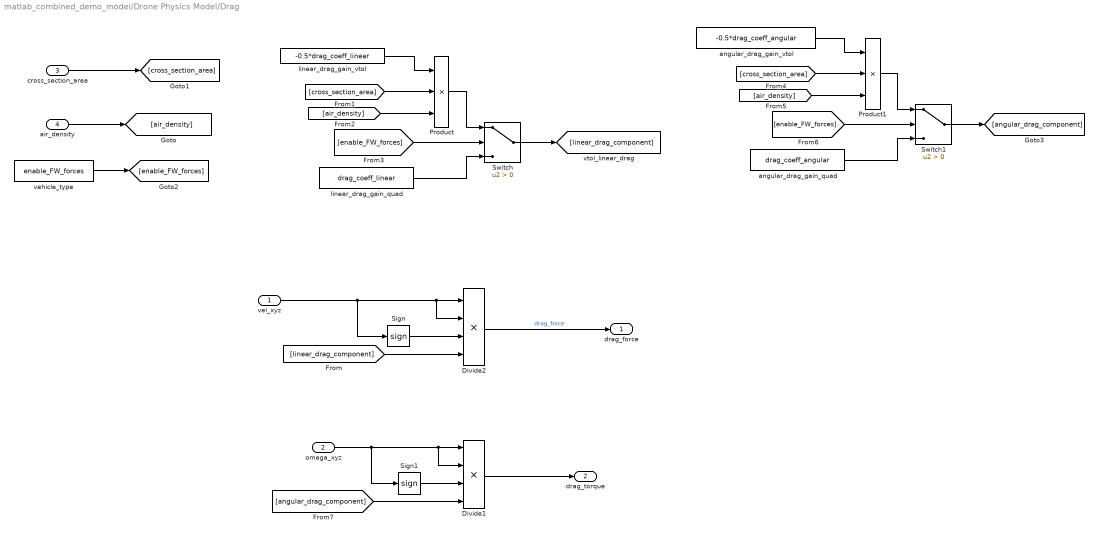
== system matlab_combined_demo_model/Drone Physics Model/Drag ==
  vel_xyz : Inport
  omega_xyz : Inport  Port=2
  cross_section_area : Inport  Port=3
  air_density : Inport  Port=4
  Divide1 : Product  Inputs=****
  Divide2 : Product  Inputs=****
  Product : Product  Inputs=3
  Product1 : Product  Inputs=3
  Sign : Signum
  Sign1 : Signum
  Switch : Switch  Criteria=u2 > Threshold  SaturateOnIntegerOverflow=off  InputSameDT=off
  Switch1 : Switch  Criteria=u2 > Threshold  SaturateOnIntegerOverflow=off  InputSameDT=off
  angular_drag_gain_quad : Constant  Value=drag_coeff_angular
  angular_drag_gain_vtol : Constant  Value=-0.5*drag_coeff_angular
  linear_drag_gain_quad : Constant  Value=drag_coeff_linear  VectorParams1D=off
  linear_drag_gain_vtol : Constant  Value=-0.5*drag_coeff_linear
  vehicle_type : Constant  Value=enable_FW_forces
  drag_force : Outport
  drag_torque : Outport  Port=2
  wires:
  vel_xyz/1 -> Sign/1, Divide2/2, Divide2/1
  Divide2/1 -> drag_force/1  "drag_force"
  Sign/1 -> Divide2/3
  Divide1/1 -> drag_torque/1
  omega_xyz/1 -> Divide1/2, Divide1/1, Sign1/1
  Sign1/1 -> Divide1/3
  [cross_section_area] -> Product/2
  linear_drag_gain_vtol/1 -> Product/1
  Product/1 -> Switch/1
  Switch/1 -> [linear_drag_component]
  linear_drag_gain_quad/1 -> Switch/3
  [enable_FW_forces] -> Switch/2
  [linear_drag_component] -> Divide2/4
  air_density/1 -> [air_density]
  cross_section_area/1 -> [cross_section_area]
  [air_density] -> Product/3
  vehicle_type/1 -> [enable_FW_forces]
  [cross_section_area] -> Product1/2
  [air_density] -> Product1/3
  angular_drag_gain_quad/1 -> Switch1/3
  Product1/1 -> Switch1/1
  [enable_FW_forces] -> Switch1/2
  angular_drag_gain_vtol/1 -> Product1/1
  Switch1/1 -> [angular_drag_component]
  [angular_drag_component] -> Divide1/4

== system matlab_combined_demo_model/Drone Physics Model/GravityForce ==
  gravity_z : Inport
  mass : Inport  Port=2
  Constant : Constant  Value=0
  Mux4 : Mux  Inputs=3
  Product : Product
  f_gravity_xyz : Outport
  wires:
  Constant/1 -> Mux4/2, Mux4/1
  Product/1 -> Mux4/3  "f_gravity"
  gravity_z/1 -> Product/1
  mass/1 -> Product/2
  Mux4/1 -> f_gravity_xyz/1  "f_gravity"

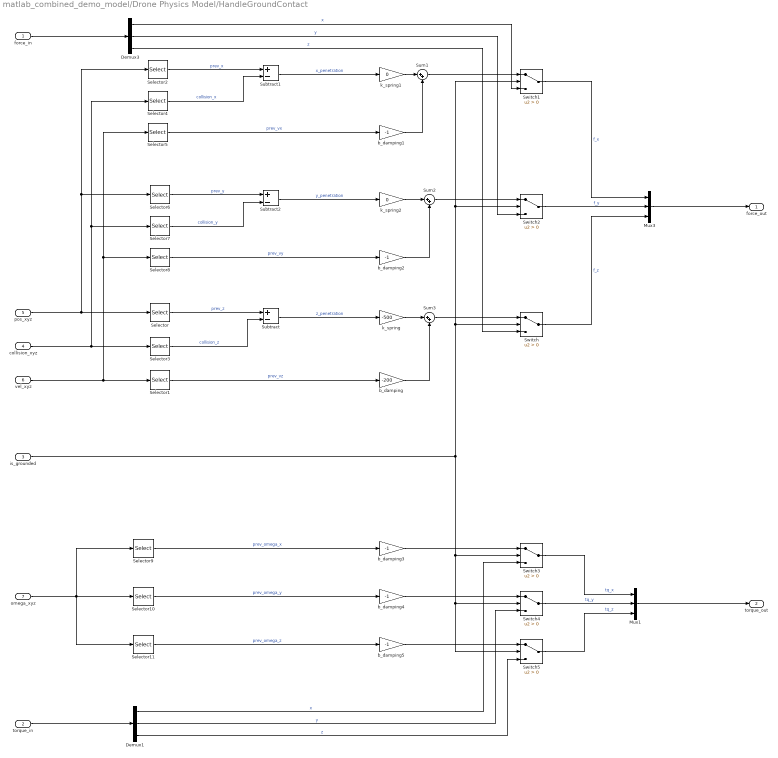
== system matlab_combined_demo_model/Drone Physics Model/HandleGroundContact ==
  force_in : Inport
  torque_in : Inport  Port=2
  is_grounded : Inport  Port=3
  collision_xyz : Inport  Port=4
  pos_xyz : Inport  Port=5
  vel_xyz : Inport  Port=6
  omega_xyz : Inport  Port=7
  Demux1 : Demux  Outputs=3
  Demux3 : Demux  Outputs=3
  Mux1 : Mux  Inputs=3
  Mux3 : Mux  Inputs=3
  Selector{,1,3,11} (4 alike) : Selector  InputPortWidth=3  IndexOptions=Index vector (dialog)  Indices=[3]  OutputSizes=1
  Selector{6..8,10} (4 alike) : Selector  InputPortWidth=3  IndexOptions=Index vector (dialog)  Indices=[2]  OutputSizes=1
  Selector{2,4..5,9} (4 alike) : Selector  InputPortWidth=3  IndexOptions=Index vector (dialog)  Indices=[1]  OutputSizes=1
  Subtract : Sum  Inputs=+-
  Subtract1 : Sum  Inputs=+-
  Subtract2 : Sum  Inputs=+-
  Sum1 : Sum  Inputs=|++
  Sum2 : Sum  Inputs=|++
  Sum3 : Sum  Inputs=|++
  Switch{,1..5} (6 alike) : Switch  Criteria=u2 > Threshold  SaturateOnIntegerOverflow=off  InputSameDT=off
  b_damping : Gain  Gain=-200
  b_damping{1..5} (5 alike) : Gain  Gain=-1
  k_spring : Gain  Gain=-500
  k_spring1 : Gain  Gain=0
  k_spring2 : Gain  Gain=0
  force_out : Outport
  torque_out : Outport  Port=2
  wires:
  Selector/1 -> Subtract/1  "prev_z"
  Subtract/1 -> k_spring/1  "z_penetration"
  Selector1/1 -> b_damping/1  "prev_vz"
  is_grounded/1 -> Switch3/2, Switch5/2, Switch4/2, Switch1/2, Switch2/2, Switch/2
  Sum3/1 -> Switch/1
  k_spring/1 -> Sum3/1
  b_damping/1 -> Sum3/2
  pos_xyz/1 -> Selector6/1, Selector2/1, Selector/1
  collision_xyz/1 -> Selector7/1, Selector4/1, Selector3/1
  Switch/1 -> Mux3/3  "f_z"
  vel_xyz/1 -> Selector8/1, Selector5/1, Selector1/1
  Switch2/1 -> Mux3/2  "f_y"
  Subtract1/1 -> k_spring1/1  "x_penetration"
  b_damping1/1 -> Sum1/2
  k_spring1/1 -> Sum1/1
  Sum1/1 -> Switch1/1
  Switch1/1 -> Mux3/1  "f_x"
  Selector3/1 -> Subtract/2  "collision_z"
  Selector5/1 -> b_damping1/1  "prev_vx"
  Selector2/1 -> Subtract1/1  "prev_x"
  Selector4/1 -> Subtract1/2  "collision_x"
  b_damping2/1 -> Sum2/2
  k_spring2/1 -> Sum2/1
  Selector8/1 -> b_damping2/1  "prev_vy"
  Subtract2/1 -> k_spring2/1  "y_penetration"
  Selector6/1 -> Subtract2/1  "prev_y"
  Sum2/1 -> Switch2/1
  Selector7/1 -> Subtract2/2  "collision_y"
  Switch3/1 -> Mux1/1  "tq_x"
  b_damping3/1 -> Switch3/1
  omega_xyz/1 -> Selector9/1, Selector11/1, Selector10/1
  Selector9/1 -> b_damping3/1  "prev_omega_x"
  Selector10/1 -> b_damping4/1  "prev_omega_y"
  Selector11/1 -> b_damping5/1  "prev_omega_z"
  Switch4/1 -> Mux1/2  "tq_y"
  b_damping4/1 -> Switch4/1
  b_damping5/1 -> Switch5/1
  Switch5/1 -> Mux1/3  "tq_z"
  Mux3/1 -> force_out/1
  force_in/1 -> Demux3/1
  Demux3/1 -> Switch1/3  "x"
  Demux3/2 -> Switch2/3  "y"
  Demux3/3 -> Switch/3  "z"
  torque_in/1 -> Demux1/1
  Demux1/1 -> Switch3/3  "x"
  Demux1/2 -> Switch4/3  "y"
  Demux1/3 -> Switch5/3  "z"
  Mux1/1 -> torque_out/1

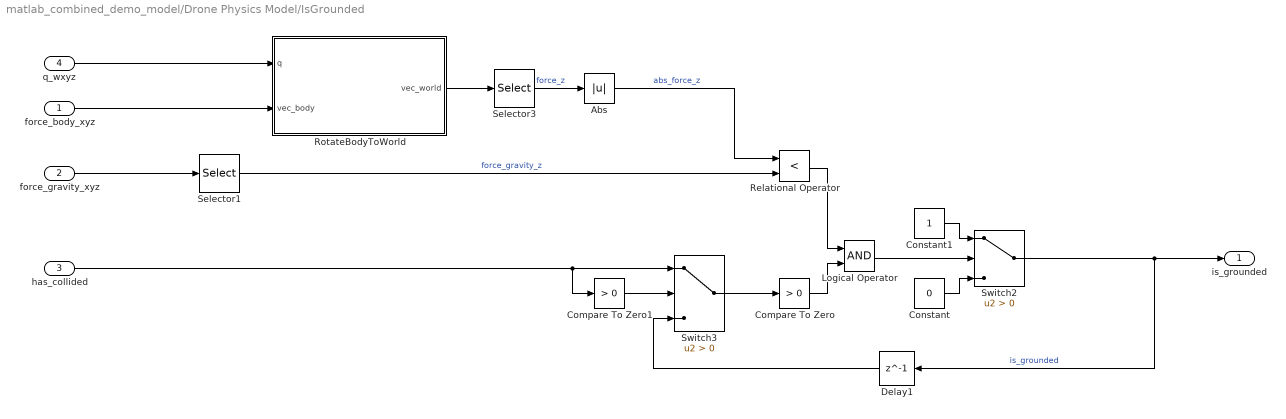
== system matlab_combined_demo_model/Drone Physics Model/IsGrounded ==
  force_body_xyz : Inport
  force_gravity_xyz : Inport  Port=2
  has_collided : Inport  Port=3
  q_wxyz : Inport  Port=4
  Abs : Abs  SaturateOnIntegerOverflow=off
  Compare To Zero : simulink/Logic and Bit Operations/Compare To Zero  relop=>  OutDataTypeStr=boolean
  Compare To Zero1 : simulink/Logic and Bit Operations/Compare To Zero  relop=>  OutDataTypeStr=boolean
  Constant : Constant  Value=0
  Constant1 : Constant
  Delay1 : Delay  DelayLength=1  InitialCondition=0
  Logical Operator : Logic  AllPortsSameDT=off  OutDataTypeStr=boolean
  Relational Operator : RelationalOperator  Operator=<  OutDataTypeStr=boolean  RndMeth=Simplest  InputSameDT=off
  RotateBodyToWorld : Subsystem
  Selector1 : Selector  InputPortWidth=3  IndexOptions=Index vector (dialog)  Indices=[3]  OutputSizes=1
  Selector3 : Selector  InputPortWidth=3  IndexOptions=Index vector (dialog)  Indices=[3]  OutputSizes=1
  Switch2 : Switch  Criteria=u2 > Threshold  SaturateOnIntegerOverflow=off  InputSameDT=off
  Switch3 : Switch  Criteria=u2 > Threshold  SaturateOnIntegerOverflow=off  InputSameDT=off
  is_grounded : Outport
  wires:
  Constant/1 -> Switch2/3
  has_collided/1 -> Compare To Zero1/1, Switch3/1
  Logical Operator/1 -> Switch2/2
  Switch3/1 -> Compare To Zero/1
  Switch2/1 -> is_grounded/1, Delay1/1  "is_grounded"
  Compare To Zero1/1 -> Switch3/2
  Relational Operator/1 -> Logical Operator/1
  Delay1/1 -> Switch3/3
  Constant1/1 -> Switch2/1
  Abs/1 -> Relational Operator/1  "abs_force_z"
  Compare To Zero/1 -> Logical Operator/2
  Selector1/1 -> Relational Operator/2  "force_gravity_z"
  force_body_xyz/1 -> RotateBodyToWorld/2(vec_body)
  force_gravity_xyz/1 -> Selector1/1
  RotateBodyToWorld/1(vec_world) -> Selector3/1
  q_wxyz/1 -> RotateBodyToWorld/1(q)
  Selector3/1 -> Abs/1  "force_z"

== system matlab_combined_demo_model/Drone Physics Model/RotateBodyToWorld ==
  q : Inport
  vec_body : Inport  Port=2
  Quaternion Inverse : aerolibutil/Quaternion Inverse
  Quaternion Rotation : aerolibutil/Quaternion Rotation
  vec_world : Outport
  wires:
  Quaternion Rotation/1 -> vec_world/1
  Quaternion Inverse/1 -> Quaternion Rotation/1
  q/1 -> Quaternion Inverse/1
  vec_body/1 -> Quaternion Rotation/2

== system matlab_combined_demo_model/Drone Physics Model/RotateBodyToWorld2 ==
  DCM : Inport
  vec_body : Inport  Port=2
  Product1 : Product  Multiplication=Matrix(*)
  Reshape1 : Reshape  OutputDimensionality=Column vector (2-D)
  Reshape2 : Reshape
  Transpose : matrix_library/Transpose
  vec_earth : Outport
  wires:
  Transpose/1 -> Product1/1
  DCM/1 -> Transpose/1
  Reshape2/1 -> vec_earth/1
  Reshape1/1 -> Product1/2
  Product1/1 -> Reshape2/1
  vec_body/1 -> Reshape1/1

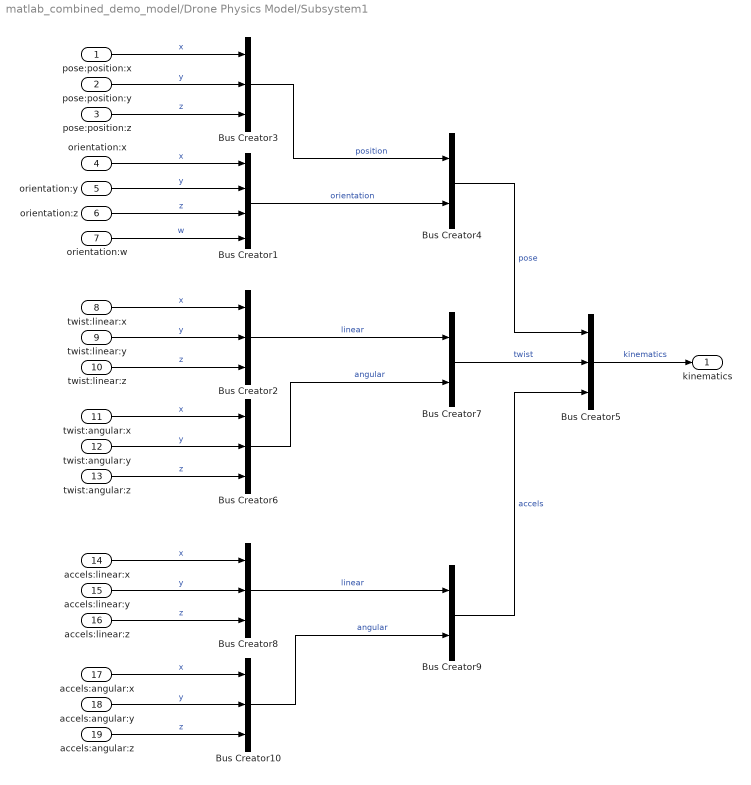
== system matlab_combined_demo_model/Drone Physics Model/Subsystem1 ==
  pose:position:x : Inport
  pose:position:y : Inport  Port=2
  pose:position:z : Inport  Port=3
  orientation:x : Inport  Port=4
  orientation:y : Inport  Port=5
  orientation:z : Inport  Port=6
  orientation:w : Inport  Port=7
  twist:linear:x : Inport  Port=8
  twist:linear:y : Inport  Port=9
  twist:linear:z : Inport  Port=10
  twist:angular:x : Inport  Port=11
  twist:angular:y : Inport  Port=12
  twist:angular:z : Inport  Port=13
  accels:linear:x : Inport  Port=14
  accels:linear:y : Inport  Port=15
  accels:linear:z : Inport  Port=16
  accels:angular:x : Inport  Port=17
  accels:angular:y : Inport  Port=18
  accels:angular:z : Inport  Port=19
  Bus Creator1 : BusCreator  Inputs=4
  Bus Creator{2..3,5..6,8,10} (6 alike) : BusCreator  Inputs=3
  Bus Creator4 : BusCreator  Inputs=2
  Bus Creator7 : BusCreator  Inputs=2
  Bus Creator9 : BusCreator  Inputs=2
  kinematics : Outport
  wires:
  Bus Creator1/1 -> Bus Creator4/2  "orientation"
  Bus Creator4/1 -> Bus Creator5/1  "pose"
  Bus Creator7/1 -> Bus Creator5/2  "twist"
  Bus Creator10/1 -> Bus Creator9/2  "angular"
  orientation:y/1 -> Bus Creator1/2  "y"
  Bus Creator2/1 -> Bus Creator7/1  "linear"
  Bus Creator3/1 -> Bus Creator4/1  "position"
  Bus Creator6/1 -> Bus Creator7/2  "angular"
  Bus Creator8/1 -> Bus Creator9/1  "linear"
  Bus Creator9/1 -> Bus Creator5/3  "accels"
  Bus Creator5/1 -> kinematics/1  "kinematics"
  accels:linear:x/1 -> Bus Creator8/1  "x"
  twist:angular:x/1 -> Bus Creator6/1  "x"
  twist:angular:z/1 -> Bus Creator6/3  "z"
  pose:position:z/1 -> Bus Creator3/3  "z"
  twist:linear:y/1 -> Bus Creator2/2  "y"
  twist:linear:x/1 -> Bus Creator2/1  "x"
  orientation:w/1 -> Bus Creator1/4  "w"
  accels:linear:z/1 -> Bus Creator8/3  "z"
  pose:position:y/1 -> Bus Creator3/2  "y"
  pose:position:x/1 -> Bus Creator3/1  "x"
  orientation:z/1 -> Bus Creator1/3  "z"
  twist:angular:y/1 -> Bus Creator6/2  "y"
  accels:linear:y/1 -> Bus Creator8/2  "y"
  accels:angular:y/1 -> Bus Creator10/2  "y"
  accels:angular:x/1 -> Bus Creator10/1  "x"
  accels:angular:z/1 -> Bus Creator10/3  "z"
  orientation:x/1 -> Bus Creator1/1  "x"
  twist:linear:z/1 -> Bus Creator2/3  "z"

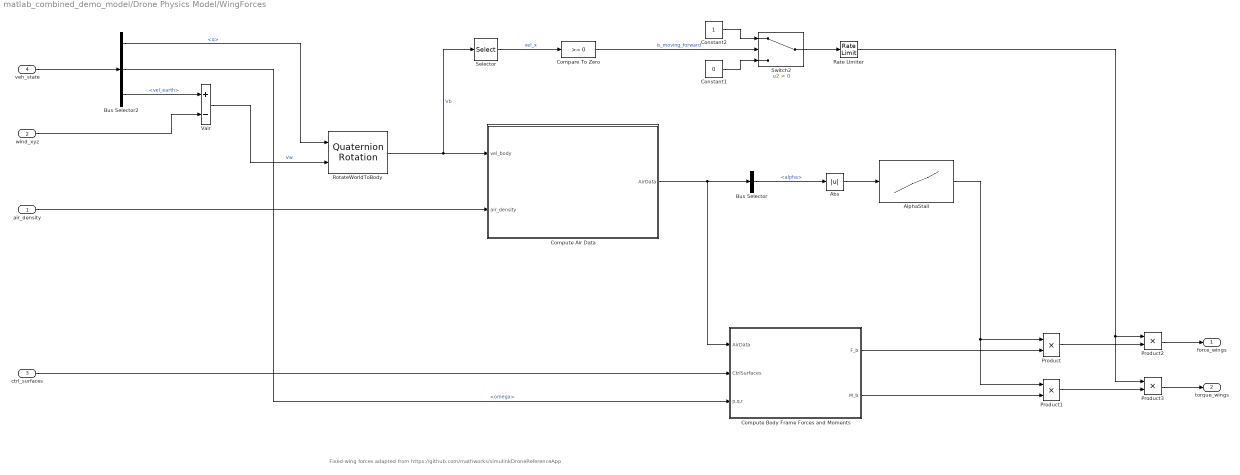
== system matlab_combined_demo_model/Drone Physics Model/WingForces ==
  note: Fixed-wing forces adapted from https://github.com/mathworks/simulinkDroneReferenceApp
  air_density : Inport
  wind_xyz : Inport  Port=2
  ctrl_surfaces : Inport  Port=3
  veh_state : Inport  Port=4
  Abs : Abs  SaturateOnIntegerOverflow=off
  AlphaStall : Lookup_n-D  NumberOfTableDimensions=1  BreakpointsForDimension1=[0,0.5,0.8,3.1416]  Table=[1,1,0,0]  InternalRulePriority=Speed  RndMeth=Simplest
  Bus Selector : BusSelector  OutputSignals=alpha
  Bus Selector2 : BusSelector  OutputSignals=q,omega,vel_earth
  Compare To Zero : simulink/Logic and Bit Operations/Compare To Zero  relop=>=  OutDataTypeStr=boolean
  Compute Air Data : Subsystem  TreatAsAtomicUnit=on  VariantControl=use_aerospace_blocks == 1
  Compute Body Frame Forces and Moments : Subsystem
  Constant1 : Constant  Value=0
  Constant2 : Constant
  Product{,1..3} (4 alike) : Product
  Rate Limiter : RateLimiter  RisingSlewLimit=10  FallingSlewLimit=-10  SampleTimeMode=inherited
  RotateWorldToBody : aerolibutil/Quaternion Rotation
  Selector : Selector  IndexMode=Zero-based  InputPortWidth=3  IndexOptions=Index vector (dialog)  Indices=[0]  OutputSizes=1
  Switch2 : Switch  Criteria=u2 > Threshold  SaturateOnIntegerOverflow=off  InputSameDT=off
  Vair : Sum  Inputs=+-  InputSameDT=on  SaturateOnIntegerOverflow=on  OutDataTypeStr=Inherit: Same as first input
  force_wings : Outport
  torque_wings : Outport  Port=2
  wires:
  veh_state/1 -> Bus Selector2/1
  Vair/1 -> RotateWorldToBody/2  "Vw"
  air_density/1 -> Compute Air Data/2(air_density)
  ctrl_surfaces/1 -> Compute Body Frame Forces and Moments/2(CtrlSurfaces)
  RotateWorldToBody/1 -> Selector/1, Compute Air Data/1(vel_body)  "Vb"
  Compute Air Data/1(AirData) -> Compute Body Frame Forces and Moments/1(AirData), Bus Selector/1
  Bus Selector2/1 -> RotateWorldToBody/1  "<q>"
  Bus Selector2/2 -> Compute Body Frame Forces and Moments/3(p,q,r)  "<omega>"
  Bus Selector2/3 -> Vair/1  "<vel_earth>"
  Selector/1 -> Compare To Zero/1  "vel_x"
  Product2/1 -> force_wings/1
  Product3/1 -> torque_wings/1
  Bus Selector/1 -> Abs/1  "<alpha>"
  AlphaStall/1 -> Product1/1, Product/1
  Compute Body Frame Forces and Moments/1(F_b) -> Product/2
  Compute Body Frame Forces and Moments/2(M_b) -> Product1/2
  wind_xyz/1 -> Vair/2
  Abs/1 -> AlphaStall/1
  Product/1 -> Product2/2
  Product1/1 -> Product3/2
  Switch2/1 -> Rate Limiter/1
  Constant2/1 -> Switch2/1
  Constant1/1 -> Switch2/3
  Compare To Zero/1 -> Switch2/2  "is_moving_forward"
  Rate Limiter/1 -> Product3/1, Product2/1

== system matlab_combined_demo_model/Subsystem/Accels ==
  linear : Inport
  angular : Inport  Port=2
  Mux5 : Mux  Inputs=2
  accels : Outport
  wires:
  linear/1 -> Mux5/1
  angular/1 -> Mux5/2
  Mux5/1 -> accels/1  "accels"

== system matlab_combined_demo_model/Subsystem/AccelsAngular ==
  x : Inport
  y : Inport  Port=2
  z : Inport  Port=3
  Mux : Mux  Inputs=3
  vector3 : Outport
  wires:
  Mux/1 -> vector3/1
  x/1 -> Mux/1
  y/1 -> Mux/2
  z/1 -> Mux/3

== system matlab_combined_demo_model/Subsystem/AccelsLinear ==
  x : Inport
  y : Inport  Port=2
  z : Inport  Port=3
  Mux : Mux  Inputs=3
  vector3 : Outport
  wires:
  Mux/1 -> vector3/1
  x/1 -> Mux/1
  y/1 -> Mux/2
  z/1 -> Mux/3

== system matlab_combined_demo_model/Subsystem/Kinematics ==
  pose : Inport
  twist : Inport  Port=2
  accels : Inport  Port=3
  Mux3 : Mux  Inputs=3
  kinematics : Outport
  wires:
  accels/1 -> Mux3/3
  pose/1 -> Mux3/1
  Mux3/1 -> kinematics/1  "kinematics"
  twist/1 -> Mux3/2

== system matlab_combined_demo_model/Subsystem/Orientation ==
  x : Inport
  y : Inport  Port=2
  z : Inport  Port=3
  w : Inport  Port=4
  Mux1 : Mux
  orientation : Outport
  wires:
  z/1 -> Mux1/3
  x/1 -> Mux1/1
  Mux1/1 -> orientation/1
  y/1 -> Mux1/2
  w/1 -> Mux1/4

== system matlab_combined_demo_model/Subsystem/Pose ==
  position : Inport
  orientation : Inport  Port=2
  Mux2 : Mux  Inputs=2
  pose : Outport
  wires:
  Mux2/1 -> pose/1  "pose"
  position/1 -> Mux2/1
  orientation/1 -> Mux2/2

== system matlab_combined_demo_model/Subsystem/Position ==
  x : Inport
  y : Inport  Port=2
  z : Inport  Port=3
  Mux : Mux  Inputs=3
  vector3 : Outport
  wires:
  Mux/1 -> vector3/1
  x/1 -> Mux/1
  y/1 -> Mux/2
  z/1 -> Mux/3

== system matlab_combined_demo_model/Subsystem/Twist ==
  linear : Inport
  angular : Inport  Port=2
  Mux5 : Mux  Inputs=2
  twist : Outport
  wires:
  angular/1 -> Mux5/2
  Mux5/1 -> twist/1  "twist"
  linear/1 -> Mux5/1

== system matlab_combined_demo_model/Subsystem/TwistAngular ==
  x : Inport
  y : Inport  Port=2
  z : Inport  Port=3
  Mux : Mux  Inputs=3
  vector3 : Outport
  wires:
  Mux/1 -> vector3/1
  x/1 -> Mux/1
  y/1 -> Mux/2
  z/1 -> Mux/3
